simulink model "Observer_design_for_sensorless_control"  (R2016b)
settings: Solver=ode45  StartTime=0.0  StopTime=1.5  FixedStep=0.0001  RelTol=1e-3
libraries: dsparch4 x2, simulink x1
settings Model: Creator=emilio  LastModifiedBy=danielesmn

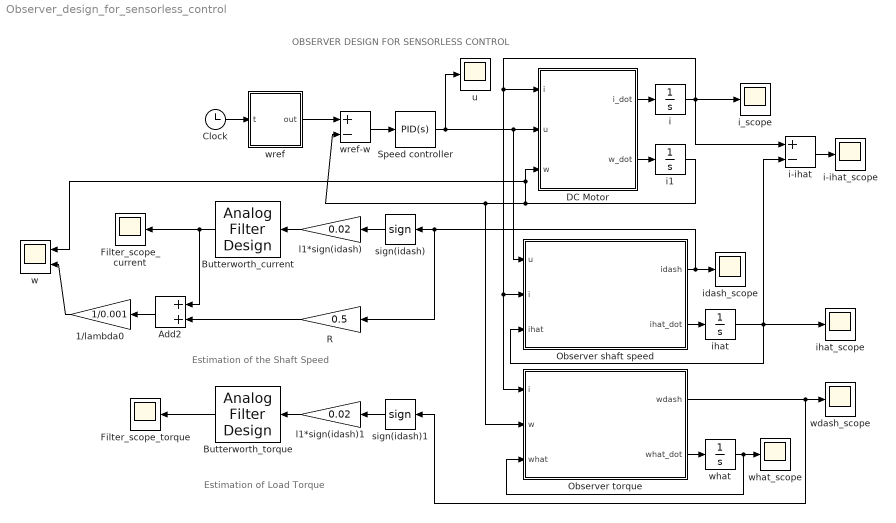
== system Observer_design_for_sensorless_control ==
  note: OBSERVER DESIGN FOR SENSORLESS CONTROL
  note: Estimation of Load Torque
  note: Estimation of the Shaft Speed
  1/lambda0 : Gain  Gain=1/0.001
  Add2 : Sum
  Butterworth_current : dsparch4/Analog Filter Design  method=Butterworth  filttype=Lowpass  N=2  Wlo=1000  Whi=80  Rp=2  Rs=40
  Butterworth_torque : dsparch4/Analog Filter Design  method=Butterworth  filttype=Lowpass  N=2  Wlo=550  Whi=80  Rp=2  Rs=40
  Clock : Clock
  DC Motor : MATLAB Function  TreatAsAtomicUnit=on
  Filter_scope_current : Scope
  Filter_scope_torque : Scope
  Observer shaft speed : MATLAB Function  TreatAsAtomicUnit=on
  Observer torque : MATLAB Function  TreatAsAtomicUnit=on
  R : Gain  Gain=0.5
  Speed controller : simulink/Continuous/PID Controller  Controller=PID  TimeDomain=Continuous-time  SampleTime=-1  IntegratorMethod=Forward Euler  FilterMethod=Forward Euler  Form=Parallel  UseFilter=on  ControllerParametersSource=internal  P=10.2296554787727  I=426.511403118429  D=0  N=176.334094339031  InitialConditionSource=internal  InitialConditionForIntegrator=0  InitialConditionForFilter=0  ExternalReset=none  LimitOutput=off  UpperSaturationLimit=inf  LowerSaturationLimit=-inf  LinearizeAsGain=on  AntiWindupMode=none  Kb=1  TrackingMode=off  Kt=1  PParamMin=[]  PParamMax=[]  IParamMin=[]  IParamMax=[]  DParamMin=[]  DParamMax=[]  NParamMin=[]  NParamMax=[]  KbParamMin=[]  KbParamMax=[]  KtParamMin=[]  KtParamMax=[]  POutMin=[]  POutMax=[]  IOutMin=[]  IOutMax=[]  DOutMin=[]  DOutMax=[]  NOutMin=[]  NOutMax=[]  KbOutMin=[]  KbOutMax=[]  KtOutMin=[]  KtOutMax=[]  IntegratorOutMin=[]  IntegratorOutMax=[]  FilterOutMin=[]  FilterOutMax=[]  SumOutMin=[]  SumOutMax=[]  SumI1OutMin=[]  SumI1OutMax=[]  SumI2OutMin=[]  SumI2OutMax=[]  SumI3OutMin=[]  SumI3OutMax=[]  SumDOutMin=[]  SumDOutMax=[]  SaturationOutMin=[]  SaturationOutMax=[]  IntegratorContinuousStateAttributes=''  IntegratorStateMustResolveToSignalObject=off  IntegratorRTWStateStorageClass=Auto  FilterContinuousStateAttributes=''  FilterStateMustResolveToSignalObject=off  FilterRTWStateStorageClass=Auto  DifferentiatorICPrevScaledInput=0  DifferentiatorOutMin=[]  DifferentiatorOutMax=[]
  i : Integrator
  i-ihat : Sum  Inputs=+-
  i-ihat_scope : Scope
  i1 : Integrator
  i_scope : Scope
  idash_scope : Scope
  ihat : Integrator  InitialCondition=0.01
  ihat_scope : Scope
  l1*sign(idash) : Gain  Gain=0.02
  l1*sign(idash)1 : Gain  Gain=0.02
  sign(idash) : Signum  ZeroCross=off
  sign(idash)1 : Signum  ZeroCross=off
  u : Scope
  w : Scope  NumInputPorts=2
  wdash_scope : Scope
  what : Integrator  InitialCondition=0.01
  what_scope : Scope
  wref : MATLAB Function  TreatAsAtomicUnit=on
  wref-w : Sum  Inputs=+-
  wires:
  Clock/1 -> wref/1(t)
  Observer shaft speed/2(ihat_dot) -> ihat/1
  DC Motor/1(i_dot) -> i/1
  i/1 -> i_scope/1, i-ihat/1, DC Motor/1(i), Observer shaft speed/2(i), Observer torque/1(i)
  DC Motor/2(w_dot) -> i1/1
  ihat/1 -> Observer shaft speed/3(ihat), i-ihat/2, ihat_scope/1
  l1*sign(idash)/1 -> Butterworth_current/1
  wref/1(out) -> wref-w/1
  i-ihat/1 -> i-ihat_scope/1
  Speed controller/1 -> DC Motor/2(u), Observer shaft speed/1(u), u/1
  wref-w/1 -> Speed controller/1
  Butterworth_current/1 -> Filter_scope_current/1, Add2/1
  Observer shaft speed/1(idash) -> R/1, sign(idash)/1, idash_scope/1
  sign(idash)/1 -> l1*sign(idash)/1
  1/lambda0/1 -> w/2
  i1/1 -> wref-w/2, Observer torque/2(w), w/1, DC Motor/3(w)
  R/1 -> Add2/2
  Add2/1 -> 1/lambda0/1
  Observer torque/2(what_dot) -> what/1
  what/1 -> what_scope/1, Observer torque/3(what)
  l1*sign(idash)1/1 -> Butterworth_torque/1
  Butterworth_torque/1 -> Filter_scope_torque/1
  sign(idash)1/1 -> l1*sign(idash)1/1
  Observer torque/1(wdash) -> wdash_scope/1, sign(idash)1/1

== matlab function Observer_design_for_sensorless_control/Observer shaft speed ==
  data: idash output; u input; i input; ihat_dot output; ihat input
function [idash, ihat_dot] = ObsCurrent(u, i, ihat)

L = 0.001;        %Armature inductance (H)
R = 0.6;          %Armature resistance (Ohm)

l1 = 0.02;        %Observer gain

idash = ihat - i;
ihat_dot = (u - R*ihat - l1*sign(idash))/L;

== matlab function Observer_design_for_sensorless_control/Observer torque ==
  data: i input; wdash output; w input; what_dot output; what input
function [wdash, what_dot] = ObsTorque(i, w, what)

kt = 0.008;       %Torque constant (Nm/A)
J = 0.001;        %Inertia of the motor rotor (Kg*m^2)

l2 = 0.02;        %Observer gain

wdash = what - w;
what_dot = (kt*i - l2*sign(wdash))/J;

== matlab function Observer_design_for_sensorless_control/DC Motor ==
  data: i input; u input; i_dot output; w input; w_dot output
function [i_dot, w_dot] = Dc_Motor(i, u, w) % i: armature current w: shaft speed

%% Model of the DC Motor

L = 0.001;        %Armature inductance (H)
R = 0.5;          %Armature resistance (Ohm)
kt = 0.008;       %Torque constant (Nm/A)
J = 0.001;        %Inertia of the motor rotor (Kg*m^2)
B = 0.01;         %Coefficient of viscous friction (Nm*s/rad)
lambda0 = 0.001;  %Back electromotive force (EMF) constant (V*s/rad)

tauL = B*w;        %Load torque

i_dot = u/L - R/L*i - lambda0/L*w;      %Electrical part model
w_dot = (kt*i - tauL)/J;              %Mechanical part model

== matlab function Observer_design_for_sensorless_control/wref ==
  data: t input; out output
function out = input(t)

if t < 0.5 || t>1
    out = -1;
else
    out = 1;
end
